simulink model "P702_NI_SoftECU"  (R2019a)
settings: Solver=ode1  StartTime=0.0  StopTime=Inf  FixedStep=0.001  RelTol=1e-3  EnableMultiTasking=on
PreLoadFcn:
  | run '.\VeriStand_BlockSet\NIVeriStandAddPaths.m'
undefined symbols (not defined in the file or in its folder): magnitude
libraries: simulink x83, simulink_extras x1
(part 74 of 76)

== system P702_NI_SoftECU/Output/Subsystem2/CAN_Signal/GWM/Other_GWMTx/Battery_Mgmt_24V_FD1 ==
  BattULo24Soc_Pc_Actl : Constant  Value=0
  BattULo24State_D_Qlty : Constant  Value=0
  BattULo24_Ah_DeltaRide : Constant  Value=0
  BattULo24_B_Falt : Constant  Value=0
  BattULo24_I_Actl : Constant  Value=0
  bus_creator : BusCreator  Inputs=5
  out_port : Outport
  wires:
  bus_creator/1 -> out_port/1  "Subsystem2"
  BattULo24Soc_Pc_Actl/1 -> bus_creator/1  "BattULo24Soc_Pc_Actl"
  BattULo24State_D_Qlty/1 -> bus_creator/2  "BattULo24State_D_Qlty"
  BattULo24_Ah_DeltaRide/1 -> bus_creator/3  "BattULo24_Ah_DeltaRide"
  BattULo24_B_Falt/1 -> bus_creator/4  "BattULo24_B_Falt"
  BattULo24_I_Actl/1 -> bus_creator/5  "BattULo24_I_Actl"

== system P702_NI_SoftECU/Output/Subsystem2/CAN_Signal/GWM/Other_GWMTx/Battery_Mgmt_2_FD1 ==
  BattULoChrg_D_Rq : Constant  Value=0
  BattULoSrvc_T_Actl : Constant  Value=0
  Batt_Crit_SoC_B : Constant  Value=0
  Batt_Lo_SoC_B : Constant  Value=0
  ChargeMode : Constant  Value=0
  EngStrtInhbt_B_RqBatt : Constant  Value=0
  IdleSpeedIncrease_El : Constant  Value=0
  PeriodicElLoad_B_Stat : Constant  Value=0
  PwSysULoFalt_D_Stat : Constant  Value=0
  Shed_Drain_Eng_Off_B : Constant  Value=0
  Shed_Feature_Group_ID : Constant  Value=0
  Shed_Level_Req : Constant  Value=0
  Shed_T_Eng_Off_B : Constant  Value=0
  ULoRgenTestMde_B_Rq : Constant  Value=0
  bus_creator : BusCreator  Inputs=14
  out_port : Outport
  wires:
  bus_creator/1 -> out_port/1  "Subsystem2"
  BattULoChrg_D_Rq/1 -> bus_creator/1  "BattULoChrg_D_Rq"
  BattULoSrvc_T_Actl/1 -> bus_creator/2  "BattULoSrvc_T_Actl"
  Batt_Crit_SoC_B/1 -> bus_creator/3  "Batt_Crit_SoC_B"
  Batt_Lo_SoC_B/1 -> bus_creator/4  "Batt_Lo_SoC_B"
  ChargeMode/1 -> bus_creator/5  "ChargeMode"
  EngStrtInhbt_B_RqBatt/1 -> bus_creator/6  "EngStrtInhbt_B_RqBatt"
  IdleSpeedIncrease_El/1 -> bus_creator/7  "IdleSpeedIncrease_El"
  PeriodicElLoad_B_Stat/1 -> bus_creator/8  "PeriodicElLoad_B_Stat"
  PwSysULoFalt_D_Stat/1 -> bus_creator/9  "PwSysULoFalt_D_Stat"
  Shed_Drain_Eng_Off_B/1 -> bus_creator/10  "Shed_Drain_Eng_Off_B"
  Shed_Feature_Group_ID/1 -> bus_creator/11  "Shed_Feature_Group_ID"
  Shed_Level_Req/1 -> bus_creator/12  "Shed_Level_Req"
  Shed_T_Eng_Off_B/1 -> bus_creator/13  "Shed_T_Eng_Off_B"
  ULoRgenTestMde_B_Rq/1 -> bus_creator/14  "ULoRgenTestMde_B_Rq"

== system P702_NI_SoftECU/Output/Subsystem2/CAN_Signal/GWM/Other_GWMTx/Battery_Mgmt_3_FD1 ==
  BSBattQCapAh : Constant  Value=0
  BSBattQDeltaRideAh : Constant  Value=0
  BSBattSOC : Constant  Value=0
  BSFault : Constant  Value=0
  BattULo2_Te_Actl : Constant  Value=0
  BattULoChrg_URate_RqMx : Constant  Value=0
  BattULoChrg_U_RqMn : Constant  Value=0
  BattULoChrg_U_RqMx : Constant  Value=0
  BattULoState_D_Qlty : Constant  Value=0
  bus_creator : BusCreator  Inputs=9
  out_port : Outport
  wires:
  bus_creator/1 -> out_port/1  "Subsystem2"
  BSBattQCapAh/1 -> bus_creator/1  "BSBattQCapAh"
  BSBattQDeltaRideAh/1 -> bus_creator/2  "BSBattQDeltaRideAh"
  BSBattSOC/1 -> bus_creator/3  "BSBattSOC"
  BSFault/1 -> bus_creator/4  "BSFault"
  BattULo2_Te_Actl/1 -> bus_creator/5  "BattULo2_Te_Actl"
  BattULoChrg_URate_RqMx/1 -> bus_creator/6  "BattULoChrg_URate_RqMx"
  BattULoChrg_U_RqMn/1 -> bus_creator/7  "BattULoChrg_U_RqMn"
  BattULoChrg_U_RqMx/1 -> bus_creator/8  "BattULoChrg_U_RqMx"
  BattULoState_D_Qlty/1 -> bus_creator/9  "BattULoState_D_Qlty"

== system P702_NI_SoftECU/Output/Subsystem2/CAN_Signal/GWM/Other_GWMTx/Battery_Mgmt_4_FD1 ==
  BattULoAuxSoc_Pc_Actl : Constant  Value=0
  BattULoAux_B_Falt : Constant  Value=0
  BattULoAux_D_Qlty : Constant  Value=0
  BattULoAux_I_Actl : Constant  Value=0
  BattULoAux_U_Actl : Constant  Value=0
  BattULoCrnkBelt_U_Pred : Constant  Value=0
  BattULoCrnkStrt_U_Pred : Constant  Value=0
  bus_creator : BusCreator  Inputs=7
  out_port : Outport
  wires:
  bus_creator/1 -> out_port/1  "Subsystem2"
  BattULoAuxSoc_Pc_Actl/1 -> bus_creator/1  "BattULoAuxSoc_Pc_Actl"
  BattULoAux_B_Falt/1 -> bus_creator/2  "BattULoAux_B_Falt"
  BattULoAux_D_Qlty/1 -> bus_creator/3  "BattULoAux_D_Qlty"
  BattULoAux_I_Actl/1 -> bus_creator/4  "BattULoAux_I_Actl"
  BattULoAux_U_Actl/1 -> bus_creator/5  "BattULoAux_U_Actl"
  BattULoCrnkBelt_U_Pred/1 -> bus_creator/6  "BattULoCrnkBelt_U_Pred"
  BattULoCrnkStrt_U_Pred/1 -> bus_creator/7  "BattULoCrnkStrt_U_Pred"

== system P702_NI_SoftECU/Output/Subsystem2/CAN_Signal/GWM/Other_GWMTx/Battery_Traction_1_FD1 ==
  BattTracMil_D_Rq : Constant  Value=0
  BattTracOffFst_D_Actl : Constant  Value=0
  BattTracOff_B_Actl : Constant  Value=0
  BattTrac_I_Actl : Constant  Value=0
  BattTrac_U_Actl : Constant  Value=0
  BattTrac_U_LimHi : Constant  Value=0
  BattTrac_U_LimLo : Constant  Value=0
  VehStrtInhbt_B_RqBatt : Constant  Value=0
  bus_creator : BusCreator  Inputs=8
  out_port : Outport
  wires:
  bus_creator/1 -> out_port/1  "Subsystem2"
  BattTracMil_D_Rq/1 -> bus_creator/1  "BattTracMil_D_Rq"
  BattTracOffFst_D_Actl/1 -> bus_creator/2  "BattTracOffFst_D_Actl"
  BattTracOff_B_Actl/1 -> bus_creator/3  "BattTracOff_B_Actl"
  BattTrac_I_Actl/1 -> bus_creator/4  "BattTrac_I_Actl"
  BattTrac_U_Actl/1 -> bus_creator/5  "BattTrac_U_Actl"
  BattTrac_U_LimHi/1 -> bus_creator/6  "BattTrac_U_LimHi"
  BattTrac_U_LimLo/1 -> bus_creator/7  "BattTrac_U_LimLo"
  VehStrtInhbt_B_RqBatt/1 -> bus_creator/8  "VehStrtInhbt_B_RqBatt"

== system P702_NI_SoftECU/Output/Subsystem2/CAN_Signal/GWM/Other_GWMTx/Battery_Traction_3_FD1 ==
  BattTracClnt_Te_Actl : Constant  Value=0
  BattTracSoc_Pc_LimHi : Constant  Value=0
  BattTracSoc_Pc_LimLo : Constant  Value=0
  BattTracSoc_Pc_MnPrtct : Constant  Value=0
  BattTracSoc_Pc_MxPrtct : Constant  Value=0
  BattTracSrvcRqd_B_Rq : Constant  Value=0
  BattTracWarnLamp_B_Rq : Constant  Value=0
  bus_creator : BusCreator  Inputs=7
  out_port : Outport
  wires:
  bus_creator/1 -> out_port/1  "Subsystem2"
  BattTracClnt_Te_Actl/1 -> bus_creator/1  "BattTracClnt_Te_Actl"
  BattTracSoc_Pc_LimHi/1 -> bus_creator/2  "BattTracSoc_Pc_LimHi"
  BattTracSoc_Pc_LimLo/1 -> bus_creator/3  "BattTracSoc_Pc_LimLo"
  BattTracSoc_Pc_MnPrtct/1 -> bus_creator/4  "BattTracSoc_Pc_MnPrtct"
  BattTracSoc_Pc_MxPrtct/1 -> bus_creator/5  "BattTracSoc_Pc_MxPrtct"
  BattTracSrvcRqd_B_Rq/1 -> bus_creator/6  "BattTracSrvcRqd_B_Rq"
  BattTracWarnLamp_B_Rq/1 -> bus_creator/7  "BattTracWarnLamp_B_Rq"

== system P702_NI_SoftECU/Output/Subsystem2/CAN_Signal/GWM/Other_GWMTx/Battery_Traction_4_FD1 ==
  BattTracDiagClr_B_Rq : Constant  Value=0
  BattTracSoc2_Pc_Actl : Constant  Value=0
  BattTrac_Te_Actl : Constant  Value=0
  bus_creator : BusCreator  Inputs=3
  out_port : Outport
  wires:
  bus_creator/1 -> out_port/1  "Subsystem2"
  BattTracDiagClr_B_Rq/1 -> bus_creator/1  "BattTracDiagClr_B_Rq"
  BattTracSoc2_Pc_Actl/1 -> bus_creator/2  "BattTracSoc2_Pc_Actl"
  BattTrac_Te_Actl/1 -> bus_creator/3  "BattTrac_Te_Actl"

== system P702_NI_SoftECU/Output/Subsystem2/CAN_Signal/GWM/Other_GWMTx/Battery_Traction_5_FD1 ==
  BattTrac2_Pw_ChrgInst : Constant  Value=0
  BattTrac2_Pw_DchrgInst : Constant  Value=0
  BattTrac2_Pw_LimChrg : Constant  Value=0
  BattTrac2_Pw_LimDchrg : Constant  Value=0
  bus_creator : BusCreator  Inputs=4
  out_port : Outport
  wires:
  bus_creator/1 -> out_port/1  "Subsystem2"
  BattTrac2_Pw_ChrgInst/1 -> bus_creator/1  "BattTrac2_Pw_ChrgInst"
  BattTrac2_Pw_DchrgInst/1 -> bus_creator/2  "BattTrac2_Pw_DchrgInst"
  BattTrac2_Pw_LimChrg/1 -> bus_creator/3  "BattTrac2_Pw_LimChrg"
  BattTrac2_Pw_LimDchrg/1 -> bus_creator/4  "BattTrac2_Pw_LimDchrg"

== system P702_NI_SoftECU/Output/Subsystem2/CAN_Signal/GWM/Other_GWMTx/Battery_Traction_6_FD1 ==
  BattTracClntPmp_D_Stat : Constant  Value=0
  BattTracCnnct_D_Cmd : Constant  Value=0
  BattTracDcdcDis_B_Rq : Constant  Value=0
  BattTracDelta_Te_Actl : Constant  Value=0
  BattTracHvilOpen_B_Stat : Constant  Value=0
  HtrnClntPump_D_Stat : Constant  Value=0
  bus_creator : BusCreator  Inputs=6
  out_port : Outport
  wires:
  bus_creator/1 -> out_port/1  "Subsystem2"
  BattTracClntPmp_D_Stat/1 -> bus_creator/1  "BattTracClntPmp_D_Stat"
  BattTracCnnct_D_Cmd/1 -> bus_creator/2  "BattTracCnnct_D_Cmd"
  BattTracDcdcDis_B_Rq/1 -> bus_creator/3  "BattTracDcdcDis_B_Rq"
  BattTracDelta_Te_Actl/1 -> bus_creator/4  "BattTracDelta_Te_Actl"
  BattTracHvilOpen_B_Stat/1 -> bus_creator/5  "BattTracHvilOpen_B_Stat"
  HtrnClntPump_D_Stat/1 -> bus_creator/6  "HtrnClntPump_D_Stat"

== system P702_NI_SoftECU/Output/Subsystem2/CAN_Signal/GWM/Other_GWMTx/BodyInfo_3_FD1 ==
  Backlit_LED_Status : Constant  Value=0
  BodySrvcRqd_B_Rq : Constant  Value=0
  CrashEvnt_D_Stat : Constant  Value=0
  Day_Night_Status : Constant  Value=0
  Delay_Accy : Constant  Value=0
  DimmingLvlEvnt_No_Actl : Constant  Value=0
  Dimming_Lvl : Constant  Value=0
  DrStatDrvErrCnt_B_Stat : Constant  Value=0
  DrStatDrv_B_Actl : Constant  Value=0
  DrStatHood_B_Actl : Constant  Value=0
  DrStatInnrTgate_B_Actl : Constant  Value=0
  DrStatPsngr_B_Actl : Constant  Value=0
  DrStatRl_B_Actl : Constant  Value=0
  DrStatRr_B_Actl : Constant  Value=0
  DrStatTgate_B_Actl : Constant  Value=0
  FogLghtFrontOn_B_Stat : Constant  Value=0
  FogLghtRearOn_B_Stat : Constant  Value=0
  FuelPmpInhbt_B_Stat : Constant  Value=0
  IgnKeyType_D_Actl : Constant  Value=0
  Ignition_Status : Constant  Value=0
  Key_In_Ignition_Stat : Constant  Value=0
  LifeCycMde_D_Actl : Constant  Value=0
  Litval : Constant  Value=0
  Parklamp_Status : Constant  Value=0
  PrkBrkActv_B_Actl : Constant  Value=0
  Remote_Start_Status : Constant  Value=0
  TurnLghtLeftOn_B_Stat : Constant  Value=0
  TurnLghtLeft_D_Rq : Constant  Value=0
  TurnLghtRightOn_B_Stat : Constant  Value=0
  TurnLghtRight_D_Rq : Constant  Value=0
  ValetMode_D_Mem : Constant  Value=0
  bus_creator : BusCreator  Inputs=31
  out_port : Outport
  wires:
  bus_creator/1 -> out_port/1  "Subsystem2"
  Backlit_LED_Status/1 -> bus_creator/1  "Backlit_LED_Status"
  BodySrvcRqd_B_Rq/1 -> bus_creator/2  "BodySrvcRqd_B_Rq"
  CrashEvnt_D_Stat/1 -> bus_creator/3  "CrashEvnt_D_Stat"
  Day_Night_Status/1 -> bus_creator/4  "Day_Night_Status"
  Delay_Accy/1 -> bus_creator/5  "Delay_Accy"
  DimmingLvlEvnt_No_Actl/1 -> bus_creator/6  "DimmingLvlEvnt_No_Actl"
  Dimming_Lvl/1 -> bus_creator/7  "Dimming_Lvl"
  DrStatDrvErrCnt_B_Stat/1 -> bus_creator/8  "DrStatDrvErrCnt_B_Stat"
  DrStatDrv_B_Actl/1 -> bus_creator/9  "DrStatDrv_B_Actl"
  DrStatHood_B_Actl/1 -> bus_creator/10  "DrStatHood_B_Actl"
  DrStatInnrTgate_B_Actl/1 -> bus_creator/11  "DrStatInnrTgate_B_Actl"
  DrStatPsngr_B_Actl/1 -> bus_creator/12  "DrStatPsngr_B_Actl"
  DrStatRl_B_Actl/1 -> bus_creator/13  "DrStatRl_B_Actl"
  DrStatRr_B_Actl/1 -> bus_creator/14  "DrStatRr_B_Actl"
  DrStatTgate_B_Actl/1 -> bus_creator/15  "DrStatTgate_B_Actl"
  FogLghtFrontOn_B_Stat/1 -> bus_creator/16  "FogLghtFrontOn_B_Stat"
  FogLghtRearOn_B_Stat/1 -> bus_creator/17  "FogLghtRearOn_B_Stat"
  FuelPmpInhbt_B_Stat/1 -> bus_creator/18  "FuelPmpInhbt_B_Stat"
  IgnKeyType_D_Actl/1 -> bus_creator/19  "IgnKeyType_D_Actl"
  Ignition_Status/1 -> bus_creator/20  "Ignition_Status"
  Key_In_Ignition_Stat/1 -> bus_creator/21  "Key_In_Ignition_Stat"
  LifeCycMde_D_Actl/1 -> bus_creator/22  "LifeCycMde_D_Actl"
  Litval/1 -> bus_creator/23  "Litval"
  Parklamp_Status/1 -> bus_creator/24  "Parklamp_Status"
  PrkBrkActv_B_Actl/1 -> bus_creator/25  "PrkBrkActv_B_Actl"
  Remote_Start_Status/1 -> bus_creator/26  "Remote_Start_Status"
  TurnLghtLeftOn_B_Stat/1 -> bus_creator/27  "TurnLghtLeftOn_B_Stat"
  TurnLghtLeft_D_Rq/1 -> bus_creator/28  "TurnLghtLeft_D_Rq"
  TurnLghtRightOn_B_Stat/1 -> bus_creator/29  "TurnLghtRightOn_B_Stat"
  TurnLghtRight_D_Rq/1 -> bus_creator/30  "TurnLghtRight_D_Rq"
  ValetMode_D_Mem/1 -> bus_creator/31  "ValetMode_D_Mem"

== system P702_NI_SoftECU/Output/Subsystem2/CAN_Signal/GWM/Other_GWMTx/Body_Info_10_FD1 ==
  GenericSwtch1_No_Actl : Constant  Value=0
  GenericSwtch2_No_Actl : Constant  Value=0
  GenericSwtch3_No_Actl : Constant  Value=0
  bus_creator : BusCreator  Inputs=3
  out_port : Outport
  wires:
  bus_creator/1 -> out_port/1  "Subsystem2"
  GenericSwtch1_No_Actl/1 -> bus_creator/1  "GenericSwtch1_No_Actl"
  GenericSwtch2_No_Actl/1 -> bus_creator/2  "GenericSwtch2_No_Actl"
  GenericSwtch3_No_Actl/1 -> bus_creator/3  "GenericSwtch3_No_Actl"

== system P702_NI_SoftECU/Output/Subsystem2/CAN_Signal/GWM/Other_GWMTx/Body_Info_4_FD1 ==
  BattULo_I_Actl : Constant  Value=0
  BattULo_U_Actl : Constant  Value=0
  BrkTrnShifLck_B_Stat : Constant  Value=0
  DcacElPw_D_Rq : Constant  Value=0
  DriverCrankingReq : Constant  Value=0
  EngOff_T_Actl : Constant  Value=0
  FuelPumpPwr_D_Stat : Constant  Value=0
  PrkLckCtlAvail_T_Stat : Constant  Value=0
  PrkLckCtlMsgTxt_D_Rq : Constant  Value=0
  PrkLckCtlTow_B_Enbl : Constant  Value=0
  PrkLckCtlUnlck_D_Stat : Constant  Value=0
  PrkLckCtl_B_Enbl : Constant  Value=0
  PtLatchActv_B_RqBcm : Constant  Value=0
  ReFuelSwtchStat_D_Actl : Constant  Value=0
  bus_creator : BusCreator  Inputs=15
  immoSecureIdleMode : Constant  Value=0
  out_port : Outport
  wires:
  bus_creator/1 -> out_port/1  "Subsystem2"
  BattULo_I_Actl/1 -> bus_creator/1  "BattULo_I_Actl"
  BattULo_U_Actl/1 -> bus_creator/2  "BattULo_U_Actl"
  BrkTrnShifLck_B_Stat/1 -> bus_creator/3  "BrkTrnShifLck_B_Stat"
  DcacElPw_D_Rq/1 -> bus_creator/4  "DcacElPw_D_Rq"
  DriverCrankingReq/1 -> bus_creator/5  "DriverCrankingReq"
  EngOff_T_Actl/1 -> bus_creator/6  "EngOff_T_Actl"
  FuelPumpPwr_D_Stat/1 -> bus_creator/7  "FuelPumpPwr_D_Stat"
  PrkLckCtlAvail_T_Stat/1 -> bus_creator/8  "PrkLckCtlAvail_T_Stat"
  PrkLckCtlMsgTxt_D_Rq/1 -> bus_creator/9  "PrkLckCtlMsgTxt_D_Rq"
  PrkLckCtlTow_B_Enbl/1 -> bus_creator/10  "PrkLckCtlTow_B_Enbl"
  PrkLckCtlUnlck_D_Stat/1 -> bus_creator/11  "PrkLckCtlUnlck_D_Stat"
  PrkLckCtl_B_Enbl/1 -> bus_creator/12  "PrkLckCtl_B_Enbl"
  PtLatchActv_B_RqBcm/1 -> bus_creator/13  "PtLatchActv_B_RqBcm"
  ReFuelSwtchStat_D_Actl/1 -> bus_creator/14  "ReFuelSwtchStat_D_Actl"
  immoSecureIdleMode/1 -> bus_creator/15  "immoSecureIdleMode"

== system P702_NI_SoftECU/Output/Subsystem2/CAN_Signal/GWM/Other_GWMTx/Body_Info_6_FD1 ==
  DrLatchMsgTxt_D_Rq : Constant  Value=0
  ElPwPoint_D_Rq : Constant  Value=0
  HeadLghtHiPrmsn_D_Stat : Constant  Value=0
  IgnPsswrdDsply_B_Rq : Constant  Value=0
  KeyAdmnTot_No_Cnt : Constant  Value=0
  KeyMykeyTot_No_Cnt : Constant  Value=0
  Keycode_Status : Constant  Value=0
  PEBackupSlot_Stats : Constant  Value=0
  PoliceIdlMde_D_Stat : Constant  Value=0
  PrmtrAlrmEvnt_D_Stat : Constant  Value=0
  PrsnlDevcChrgEnbl_B_Rq : Constant  Value=0
  SecurityMsgTxt_D_Rq : Constant  Value=0
  SteWhlLckMsgTxt_D_Rq : Constant  Value=0
  TracKeyMde_D_Stat : Constant  Value=0
  bus_creator : BusCreator  Inputs=15
  immoMsgTxt_D_Rq : Constant  Value=0
  out_port : Outport
  wires:
  bus_creator/1 -> out_port/1  "Subsystem2"
  DrLatchMsgTxt_D_Rq/1 -> bus_creator/1  "DrLatchMsgTxt_D_Rq"
  ElPwPoint_D_Rq/1 -> bus_creator/2  "ElPwPoint_D_Rq"
  HeadLghtHiPrmsn_D_Stat/1 -> bus_creator/3  "HeadLghtHiPrmsn_D_Stat"
  IgnPsswrdDsply_B_Rq/1 -> bus_creator/4  "IgnPsswrdDsply_B_Rq"
  KeyAdmnTot_No_Cnt/1 -> bus_creator/5  "KeyAdmnTot_No_Cnt"
  KeyMykeyTot_No_Cnt/1 -> bus_creator/6  "KeyMykeyTot_No_Cnt"
  Keycode_Status/1 -> bus_creator/7  "Keycode_Status"
  PEBackupSlot_Stats/1 -> bus_creator/8  "PEBackupSlot_Stats"
  PoliceIdlMde_D_Stat/1 -> bus_creator/9  "PoliceIdlMde_D_Stat"
  PrmtrAlrmEvnt_D_Stat/1 -> bus_creator/10  "PrmtrAlrmEvnt_D_Stat"
  PrsnlDevcChrgEnbl_B_Rq/1 -> bus_creator/11  "PrsnlDevcChrgEnbl_B_Rq"
  SecurityMsgTxt_D_Rq/1 -> bus_creator/12  "SecurityMsgTxt_D_Rq"
  SteWhlLckMsgTxt_D_Rq/1 -> bus_creator/13  "SteWhlLckMsgTxt_D_Rq"
  TracKeyMde_D_Stat/1 -> bus_creator/14  "TracKeyMde_D_Stat"
  immoMsgTxt_D_Rq/1 -> bus_creator/15  "immoMsgTxt_D_Rq"

== system P702_NI_SoftECU/Output/Subsystem2/CAN_Signal/GWM/Other_GWMTx/Body_Info_8_FD1 ==
  ChrgCordLck_B_Stat : Constant  Value=0
  ChrgCordResp1_No_Actl : Constant  Value=0
  ChrgCordResp2_No_Actl : Constant  Value=0
  WakeAlarm0_D_Stat : Constant  Value=0
  WakeAlarm1_D_Stat : Constant  Value=0
  WakeAlarm2_D_Stat : Constant  Value=0
  WakeAlarm3_D_Stat : Constant  Value=0
  bus_creator : BusCreator  Inputs=7
  out_port : Outport
  wires:
  bus_creator/1 -> out_port/1  "Subsystem2"
  ChrgCordLck_B_Stat/1 -> bus_creator/1  "ChrgCordLck_B_Stat"
  ChrgCordResp1_No_Actl/1 -> bus_creator/2  "ChrgCordResp1_No_Actl"
  ChrgCordResp2_No_Actl/1 -> bus_creator/3  "ChrgCordResp2_No_Actl"
  WakeAlarm0_D_Stat/1 -> bus_creator/4  "WakeAlarm0_D_Stat"
  WakeAlarm1_D_Stat/1 -> bus_creator/5  "WakeAlarm1_D_Stat"
  WakeAlarm2_D_Stat/1 -> bus_creator/6  "WakeAlarm2_D_Stat"
  WakeAlarm3_D_Stat/1 -> bus_creator/7  "WakeAlarm3_D_Stat"

== system P702_NI_SoftECU/Output/Subsystem2/CAN_Signal/GWM/Other_GWMTx/Body_Info_9_FD1 ==
  AdvStrt_D_Stat : Constant  Value=0
  CrnkInhbt_B_Stat : Constant  Value=0
  CrnkInhbt_No_Cnt : Constant  Value=0
  CrnkInhbt_No_Cs : Constant  Value=0
  DrvInCtl_B_Stat : Constant  Value=0
  EngStrtActv_B_Stat : Constant  Value=0
  EngStrt_B_Rq : Constant  Value=0
  IgnPreOffActv_B_Stat : Constant  Value=0
  StrtrMtrCtlDStat_No_Cs : Constant  Value=0
  VehOnSrc_D_Stat : Constant  Value=0
  bus_creator : BusCreator  Inputs=10
  out_port : Outport
  wires:
  bus_creator/1 -> out_port/1  "Subsystem2"
  AdvStrt_D_Stat/1 -> bus_creator/1  "AdvStrt_D_Stat"
  CrnkInhbt_B_Stat/1 -> bus_creator/2  "CrnkInhbt_B_Stat"
  CrnkInhbt_No_Cnt/1 -> bus_creator/3  "CrnkInhbt_No_Cnt"
  CrnkInhbt_No_Cs/1 -> bus_creator/4  "CrnkInhbt_No_Cs"
  DrvInCtl_B_Stat/1 -> bus_creator/5  "DrvInCtl_B_Stat"
  EngStrtActv_B_Stat/1 -> bus_creator/6  "EngStrtActv_B_Stat"
  EngStrt_B_Rq/1 -> bus_creator/7  "EngStrt_B_Rq"
  IgnPreOffActv_B_Stat/1 -> bus_creator/8  "IgnPreOffActv_B_Stat"
  StrtrMtrCtlDStat_No_Cs/1 -> bus_creator/9  "StrtrMtrCtlDStat_No_Cs"
  VehOnSrc_D_Stat/1 -> bus_creator/10  "VehOnSrc_D_Stat"

== system P702_NI_SoftECU/Output/Subsystem2/CAN_Signal/GWM/Other_GWMTx/Climate_Cntrl_Data_2_FD1 ==
  ApaSwtch_D_RqDrv : Constant  Value=0
  ApaSwtch_No_Cnt : Constant  Value=0
  CabnAmb_Te_Actl : Constant  Value=0
  CamraDefog_B_Actl : Constant  Value=0
  ClimtThrmlLoad_No_Actl : Constant  Value=0
  EcoMde_D_RqDrv : Constant  Value=0
  HvacAir_Flw_Est : Constant  Value=0
  HvacBlwrFront_D_Stat : Constant  Value=0
  HvacBlwrRear_D_Stat : Constant  Value=0
  HvacRec_Pc_Est : Constant  Value=0
  HvacRemoteStrt_N_Rq : Constant  Value=0
  TwHlGrdAsst_B_RqTrn : Constant  Value=0
  bus_creator : BusCreator  Inputs=12
  out_port : Outport
  wires:
  bus_creator/1 -> out_port/1  "Subsystem2"
  ApaSwtch_D_RqDrv/1 -> bus_creator/1  "ApaSwtch_D_RqDrv"
  ApaSwtch_No_Cnt/1 -> bus_creator/2  "ApaSwtch_No_Cnt"
  CabnAmb_Te_Actl/1 -> bus_creator/3  "CabnAmb_Te_Actl"
  CamraDefog_B_Actl/1 -> bus_creator/4  "CamraDefog_B_Actl"
  ClimtThrmlLoad_No_Actl/1 -> bus_creator/5  "ClimtThrmlLoad_No_Actl"
  EcoMde_D_RqDrv/1 -> bus_creator/6  "EcoMde_D_RqDrv"
  HvacAir_Flw_Est/1 -> bus_creator/7  "HvacAir_Flw_Est"
  HvacBlwrFront_D_Stat/1 -> bus_creator/8  "HvacBlwrFront_D_Stat"
  HvacBlwrRear_D_Stat/1 -> bus_creator/9  "HvacBlwrRear_D_Stat"
  HvacRec_Pc_Est/1 -> bus_creator/10  "HvacRec_Pc_Est"
  HvacRemoteStrt_N_Rq/1 -> bus_creator/11  "HvacRemoteStrt_N_Rq"
  TwHlGrdAsst_B_RqTrn/1 -> bus_creator/12  "TwHlGrdAsst_B_RqTrn"

== system P702_NI_SoftECU/Output/Subsystem2/CAN_Signal/GWM/Other_GWMTx/Climate_Control_Data_FD1 ==
  AutoHoldSwtch_D_Stat : Constant  Value=0
  CamraFrntBttn_D_Stat : Constant  Value=0
  CamraRearBttn_D_Stat : Constant  Value=0
  DrvSlipCtlMde_B_Rq : Constant  Value=0
  EcoInhbt_B_RqHvac : Constant  Value=0
  GlvBoxRleas_No_Actl : Constant  Value=0
  LpdbAuxBlwr_B_Rq : Constant  Value=0
  LpdbDfrstFlOn_B_Rq : Constant  Value=0
  LpdbDfrstFrOn_B_Rq : Constant  Value=0
  LpdbDfrstRearOn_B_Rq : Constant  Value=0
  LpdbHeatWiprPrk_B_Rq : Constant  Value=0
  LpdbPtc1_B_Rq : Constant  Value=0
  LpdbPtc2_B_Rq : Constant  Value=0
  LpdbPtc3_B_Rq : Constant  Value=0
  MirrorHeatOn_B_Rq : Constant  Value=0
  Outside_Air_Temp_Stat : Constant  Value=0
  PrkAidSwtch_D_RqDrv : Constant  Value=0
  PrkAidSwtch_No_Cnt : Constant  Value=0
  Remote_Start_QuietMode : Constant  Value=0
  SteWhlHeat_D_Rq : Constant  Value=0
  TrailCtlSwtch_B_Stat : Constant  Value=0
  bus_creator : BusCreator  Inputs=21
  out_port : Outport
  wires:
  bus_creator/1 -> out_port/1  "Subsystem2"
  AutoHoldSwtch_D_Stat/1 -> bus_creator/1  "AutoHoldSwtch_D_Stat"
  CamraFrntBttn_D_Stat/1 -> bus_creator/2  "CamraFrntBttn_D_Stat"
  CamraRearBttn_D_Stat/1 -> bus_creator/3  "CamraRearBttn_D_Stat"
  DrvSlipCtlMde_B_Rq/1 -> bus_creator/4  "DrvSlipCtlMde_B_Rq"
  EcoInhbt_B_RqHvac/1 -> bus_creator/5  "EcoInhbt_B_RqHvac"
  GlvBoxRleas_No_Actl/1 -> bus_creator/6  "GlvBoxRleas_No_Actl"
  LpdbAuxBlwr_B_Rq/1 -> bus_creator/7  "LpdbAuxBlwr_B_Rq"
  LpdbDfrstFlOn_B_Rq/1 -> bus_creator/8  "LpdbDfrstFlOn_B_Rq"
  LpdbDfrstFrOn_B_Rq/1 -> bus_creator/9  "LpdbDfrstFrOn_B_Rq"
  LpdbDfrstRearOn_B_Rq/1 -> bus_creator/10  "LpdbDfrstRearOn_B_Rq"
  LpdbHeatWiprPrk_B_Rq/1 -> bus_creator/11  "LpdbHeatWiprPrk_B_Rq"
  LpdbPtc1_B_Rq/1 -> bus_creator/12  "LpdbPtc1_B_Rq"
  LpdbPtc2_B_Rq/1 -> bus_creator/13  "LpdbPtc2_B_Rq"
  LpdbPtc3_B_Rq/1 -> bus_creator/14  "LpdbPtc3_B_Rq"
  MirrorHeatOn_B_Rq/1 -> bus_creator/15  "MirrorHeatOn_B_Rq"
  Outside_Air_Temp_Stat/1 -> bus_creator/16  "Outside_Air_Temp_Stat"
  PrkAidSwtch_D_RqDrv/1 -> bus_creator/17  "PrkAidSwtch_D_RqDrv"
  PrkAidSwtch_No_Cnt/1 -> bus_creator/18  "PrkAidSwtch_No_Cnt"
  Remote_Start_QuietMode/1 -> bus_creator/19  "Remote_Start_QuietMode"
  SteWhlHeat_D_Rq/1 -> bus_creator/20  "SteWhlHeat_D_Rq"
  TrailCtlSwtch_B_Stat/1 -> bus_creator/21  "TrailCtlSwtch_B_Stat"

== system P702_NI_SoftECU/Output/Subsystem2/CAN_Signal/GWM/Other_GWMTx/Cluster_Info1_FD1 ==
  AccDeny_B_RqIpc : Constant  Value=0
  AccEnbl_B_RqDrv : Constant  Value=0
  BulbChkActv_B_Stat : Constant  Value=0
  DrvPerfMde_D_Rq : Constant  Value=0
  DrvSlipCtlMde_B_Rq2 : Constant  Value=0
  DrvSlipCtlMde_D_Rq : Constant  Value=0
  EmgcyCallAsstMykey_Rq : Constant  Value=0
  EngIdlShutDown_B_RqDrv : Constant  Value=0
  EngOilLife_B_RqReset : Constant  Value=0
  Fda_B_Stat : Constant  Value=0
  FrostWarn_D_Stat : Constant  Value=0
  HsaMde_D_Rq : Constant  Value=0
  KeyTypeChngMykey_D_Rq : Constant  Value=0
  LscmbbStat_B_Actl : Constant  Value=0
  ManRgen_D_Rq : Constant  Value=0
  MetricActvTe_B_Actl : Constant  Value=0
  MetricActv_B_Actl : Constant  Value=0
  NtrlTowMdeEnbl_B_RqDrv : Constant  Value=0
  OdometerMasterValue : Constant  Value=0
  ParkDetect_Stat : Constant  Value=0
  Power_Liftgate_Mode_Cmd : Constant  Value=0
  PrkLckCtlEnbl_D_RqIpc : Constant  Value=0
  PtDrvMde_D_Rq : Constant  Value=0
  ReducedGuard_D_Rq : Constant  Value=0
  StopStrtDrvMde_D_RqMnu : Constant  Value=0
  TRAILER_BRAKE_CONFIG : Constant  Value=0
  TRLR_SWAY_CONFIG_CMD : Constant  Value=0
  TrlrBrkMde_D_Rq : Constant  Value=0
  bus_creator : BusCreator  Inputs=29
  ePRNDL_MODE : Constant  Value=0
  out_port : Outport
  wires:
  bus_creator/1 -> out_port/1  "Subsystem2"
  AccDeny_B_RqIpc/1 -> bus_creator/1  "AccDeny_B_RqIpc"
  AccEnbl_B_RqDrv/1 -> bus_creator/2  "AccEnbl_B_RqDrv"
  BulbChkActv_B_Stat/1 -> bus_creator/3  "BulbChkActv_B_Stat"
  DrvPerfMde_D_Rq/1 -> bus_creator/4  "DrvPerfMde_D_Rq"
  DrvSlipCtlMde_B_Rq2/1 -> bus_creator/5  "DrvSlipCtlMde_B_Rq2"
  DrvSlipCtlMde_D_Rq/1 -> bus_creator/6  "DrvSlipCtlMde_D_Rq"
  EmgcyCallAsstMykey_Rq/1 -> bus_creator/7  "EmgcyCallAsstMykey_Rq"
  EngIdlShutDown_B_RqDrv/1 -> bus_creator/8  "EngIdlShutDown_B_RqDrv"
  EngOilLife_B_RqReset/1 -> bus_creator/9  "EngOilLife_B_RqReset"
  Fda_B_Stat/1 -> bus_creator/10  "Fda_B_Stat"
  FrostWarn_D_Stat/1 -> bus_creator/11  "FrostWarn_D_Stat"
  HsaMde_D_Rq/1 -> bus_creator/12  "HsaMde_D_Rq"
  KeyTypeChngMykey_D_Rq/1 -> bus_creator/13  "KeyTypeChngMykey_D_Rq"
  LscmbbStat_B_Actl/1 -> bus_creator/14  "LscmbbStat_B_Actl"
  ManRgen_D_Rq/1 -> bus_creator/15  "ManRgen_D_Rq"
  MetricActvTe_B_Actl/1 -> bus_creator/16  "MetricActvTe_B_Actl"
  MetricActv_B_Actl/1 -> bus_creator/17  "MetricActv_B_Actl"
  NtrlTowMdeEnbl_B_RqDrv/1 -> bus_creator/18  "NtrlTowMdeEnbl_B_RqDrv"
  OdometerMasterValue/1 -> bus_creator/19  "OdometerMasterValue"
  ParkDetect_Stat/1 -> bus_creator/20  "ParkDetect_Stat"
  Power_Liftgate_Mode_Cmd/1 -> bus_creator/21  "Power_Liftgate_Mode_Cmd"
  PrkLckCtlEnbl_D_RqIpc/1 -> bus_creator/22  "PrkLckCtlEnbl_D_RqIpc"
  PtDrvMde_D_Rq/1 -> bus_creator/23  "PtDrvMde_D_Rq"
  ReducedGuard_D_Rq/1 -> bus_creator/24  "ReducedGuard_D_Rq"
  StopStrtDrvMde_D_RqMnu/1 -> bus_creator/25  "StopStrtDrvMde_D_RqMnu"
  TRAILER_BRAKE_CONFIG/1 -> bus_creator/26  "TRAILER_BRAKE_CONFIG"
  TRLR_SWAY_CONFIG_CMD/1 -> bus_creator/27  "TRLR_SWAY_CONFIG_CMD"
  TrlrBrkMde_D_Rq/1 -> bus_creator/28  "TrlrBrkMde_D_Rq"
  ePRNDL_MODE/1 -> bus_creator/29  "ePRNDL_MODE"

== system P702_NI_SoftECU/Output/Subsystem2/CAN_Signal/GWM/Other_GWMTx/Cluster_Info_3_FD1 ==
  AutoRgen_D_Rq : Constant  Value=0
  DISPLAY_SPEED_OFFSET : Constant  Value=0
  DISPLAY_SPEED_SCALING : Constant  Value=0
  DrvSlipCtlMde_B_RqMyKey : Constant  Value=0
  FUEL_SENSOR_NUM : Constant  Value=0
  FuelLvlActvSide_No_Raw : Constant  Value=0
  FuelLvlPssvSide_No_Raw : Constant  Value=0
  FuelLvlWarn_D_Actl : Constant  Value=0
  FuelLvl_Pc_Dsply : Constant  Value=0
  FuelSecndActv_B_Actl : Constant  Value=0
  OdoTripRx_B_Actl : Constant  Value=0
  Veh_V_CompLimMx : Constant  Value=0
  W2S_LAMP_OK : Constant  Value=0
  bus_creator : BusCreator  Inputs=13
  out_port : Outport
  wires:
  bus_creator/1 -> out_port/1  "Subsystem2"
  AutoRgen_D_Rq/1 -> bus_creator/1  "AutoRgen_D_Rq"
  DISPLAY_SPEED_OFFSET/1 -> bus_creator/2  "DISPLAY_SPEED_OFFSET"
  DISPLAY_SPEED_SCALING/1 -> bus_creator/3  "DISPLAY_SPEED_SCALING"
  DrvSlipCtlMde_B_RqMyKey/1 -> bus_creator/4  "DrvSlipCtlMde_B_RqMyKey"
  FUEL_SENSOR_NUM/1 -> bus_creator/5  "FUEL_SENSOR_NUM"
  FuelLvlActvSide_No_Raw/1 -> bus_creator/6  "FuelLvlActvSide_No_Raw"
  FuelLvlPssvSide_No_Raw/1 -> bus_creator/7  "FuelLvlPssvSide_No_Raw"
  FuelLvlWarn_D_Actl/1 -> bus_creator/8  "FuelLvlWarn_D_Actl"
  FuelLvl_Pc_Dsply/1 -> bus_creator/9  "FuelLvl_Pc_Dsply"
  FuelSecndActv_B_Actl/1 -> bus_creator/10  "FuelSecndActv_B_Actl"
  OdoTripRx_B_Actl/1 -> bus_creator/11  "OdoTripRx_B_Actl"
  Veh_V_CompLimMx/1 -> bus_creator/12  "Veh_V_CompLimMx"
  W2S_LAMP_OK/1 -> bus_creator/13  "W2S_LAMP_OK"

== system P702_NI_SoftECU/Output/Subsystem2/CAN_Signal/GWM/Other_GWMTx/Cluster_Lighting_Rq_FD1 ==
  IsaOffst_D_Rq : Constant  Value=0
  SlMde_D_Rq : Constant  Value=0
  bus_creator : BusCreator  Inputs=2
  out_port : Outport
  wires:
  bus_creator/1 -> out_port/1  "Subsystem2"
  IsaOffst_D_Rq/1 -> bus_creator/1  "IsaOffst_D_Rq"
  SlMde_D_Rq/1 -> bus_creator/2  "SlMde_D_Rq"

== system P702_NI_SoftECU/Output/Subsystem2/CAN_Signal/GWM/Other_GWMTx/Compressor_Req_FD1 ==
  ClimtCoolRear_B_Rq : Constant  Value=0
  ClimtCool_D_Rq : Constant  Value=0
  ClimtDeltaLoad_Pw_Actl : Constant  Value=0
  ClimtHeatRear_D_Rq : Constant  Value=0
  ClimtHeat_D_Rq : Constant  Value=0
  ClimtPw_B_Rq : Constant  Value=0
  HtrCorePump_B_Rq : Constant  Value=0
  HvacAirCond_B_Rq : Constant  Value=0
  HvacEvap_Te_Actl : Constant  Value=0
  HvacEvap_Te_Offst : Constant  Value=0
  HvacEvap_Te_Rq : Constant  Value=0
  HvacHtrCore_Te_Rq : Constant  Value=0
  SnowPlowMde_B_Enbl : Constant  Value=0
  StopStrtDrvMde_B_RqBtn : Constant  Value=0
  WndwFrontHeat_B_Stat : Constant  Value=0
  bus_creator : BusCreator  Inputs=15
  out_port : Outport
  wires:
  bus_creator/1 -> out_port/1  "Subsystem2"
  ClimtCoolRear_B_Rq/1 -> bus_creator/1  "ClimtCoolRear_B_Rq"
  ClimtCool_D_Rq/1 -> bus_creator/2  "ClimtCool_D_Rq"
  ClimtDeltaLoad_Pw_Actl/1 -> bus_creator/3  "ClimtDeltaLoad_Pw_Actl"
  ClimtHeatRear_D_Rq/1 -> bus_creator/4  "ClimtHeatRear_D_Rq"
  ClimtHeat_D_Rq/1 -> bus_creator/5  "ClimtHeat_D_Rq"
  ClimtPw_B_Rq/1 -> bus_creator/6  "ClimtPw_B_Rq"
  HtrCorePump_B_Rq/1 -> bus_creator/7  "HtrCorePump_B_Rq"
  HvacAirCond_B_Rq/1 -> bus_creator/8  "HvacAirCond_B_Rq"
  HvacEvap_Te_Actl/1 -> bus_creator/9  "HvacEvap_Te_Actl"
  HvacEvap_Te_Offst/1 -> bus_creator/10  "HvacEvap_Te_Offst"
  HvacEvap_Te_Rq/1 -> bus_creator/11  "HvacEvap_Te_Rq"
  HvacHtrCore_Te_Rq/1 -> bus_creator/12  "HvacHtrCore_Te_Rq"
  SnowPlowMde_B_Enbl/1 -> bus_creator/13  "SnowPlowMde_B_Enbl"
  StopStrtDrvMde_B_RqBtn/1 -> bus_creator/14  "StopStrtDrvMde_B_RqBtn"
  WndwFrontHeat_B_Stat/1 -> bus_creator/15  "WndwFrontHeat_B_Stat"

== system P702_NI_SoftECU/Output/Subsystem2/CAN_Signal/GWM/Other_GWMTx/CruiseCtrl_Strg_Data_FD1 ==
  AccButtnGapDecPress2 : Constant  Value=0
  AccButtnGapIncPress2 : Constant  Value=0
  AccButtnGpTogglePress2 : Constant  Value=0
  ActvFrontSteLck_D_Stat : Constant  Value=0
  ActvFrontSteMsgTxt_D_Rq : Constant  Value=0
  AslButtnOnOffCnclPres2 : Constant  Value=0
  AslButtnOnOffPress2 : Constant  Value=0
  CcAslButtnCnclPress2 : Constant  Value=0
  CcAslButtnCnclResPres2 : Constant  Value=0
  CcAslButtnDeny_B_Actl2 : Constant  Value=0
  CcAslButtnIndxDecPres2 : Constant  Value=0
  CcAslButtnIndxIncPres2 : Constant  Value=0
  CcAslButtnOffCnclPres2 : Constant  Value=0
  CcAslButtnOnOffCncl2 : Constant  Value=0
  CcAslButtnOnPress2 : Constant  Value=0
  CcAslButtnResDecPress2 : Constant  Value=0
  CcAslButtnResIncPress2 : Constant  Value=0
  CcAslButtnSetDecPress2 : Constant  Value=0
  CcAslButtnSetIncPress2 : Constant  Value=0
  CcAslButtnSetPress2 : Constant  Value=0
  CcAsllButtnResPress2 : Constant  Value=0
  CcButtnOffPress2 : Constant  Value=0
  CcButtnOnOffCnclPress2 : Constant  Value=0
  CcButtnOnOffPress2 : Constant  Value=0
  CcButtnOnPress2 : Constant  Value=0
  SelDrvMdeAdptSte_D_Stat : Constant  Value=0
  TjaButtnOnOffPress2 : Constant  Value=0
  bus_creator : BusCreator  Inputs=27
  out_port : Outport
  wires:
  bus_creator/1 -> out_port/1  "Subsystem2"
  AccButtnGapDecPress2/1 -> bus_creator/1  "AccButtnGapDecPress2"
  AccButtnGapIncPress2/1 -> bus_creator/2  "AccButtnGapIncPress2"
  AccButtnGpTogglePress2/1 -> bus_creator/3  "AccButtnGpTogglePress2"
  ActvFrontSteLck_D_Stat/1 -> bus_creator/4  "ActvFrontSteLck_D_Stat"
  ActvFrontSteMsgTxt_D_Rq/1 -> bus_creator/5  "ActvFrontSteMsgTxt_D_Rq"
  AslButtnOnOffCnclPres2/1 -> bus_creator/6  "AslButtnOnOffCnclPres2"
  AslButtnOnOffPress2/1 -> bus_creator/7  "AslButtnOnOffPress2"
  CcAslButtnCnclPress2/1 -> bus_creator/8  "CcAslButtnCnclPress2"
  CcAslButtnCnclResPres2/1 -> bus_creator/9  "CcAslButtnCnclResPres2"
  CcAslButtnDeny_B_Actl2/1 -> bus_creator/10  "CcAslButtnDeny_B_Actl2"
  CcAslButtnIndxDecPres2/1 -> bus_creator/11  "CcAslButtnIndxDecPres2"
  CcAslButtnIndxIncPres2/1 -> bus_creator/12  "CcAslButtnIndxIncPres2"
  CcAslButtnOffCnclPres2/1 -> bus_creator/13  "CcAslButtnOffCnclPres2"
  CcAslButtnOnOffCncl2/1 -> bus_creator/14  "CcAslButtnOnOffCncl2"
  CcAslButtnOnPress2/1 -> bus_creator/15  "CcAslButtnOnPress2"
  CcAslButtnResDecPress2/1 -> bus_creator/16  "CcAslButtnResDecPress2"
  CcAslButtnResIncPress2/1 -> bus_creator/17  "CcAslButtnResIncPress2"
  CcAslButtnSetDecPress2/1 -> bus_creator/18  "CcAslButtnSetDecPress2"
  CcAslButtnSetIncPress2/1 -> bus_creator/19  "CcAslButtnSetIncPress2"
  CcAslButtnSetPress2/1 -> bus_creator/20  "CcAslButtnSetPress2"
  CcAsllButtnResPress2/1 -> bus_creator/21  "CcAsllButtnResPress2"
  CcButtnOffPress2/1 -> bus_creator/22  "CcButtnOffPress2"
  CcButtnOnOffCnclPress2/1 -> bus_creator/23  "CcButtnOnOffCnclPress2"
  CcButtnOnOffPress2/1 -> bus_creator/24  "CcButtnOnOffPress2"
  CcButtnOnPress2/1 -> bus_creator/25  "CcButtnOnPress2"
  SelDrvMdeAdptSte_D_Stat/1 -> bus_creator/26  "SelDrvMdeAdptSte_D_Stat"
  TjaButtnOnOffPress2/1 -> bus_creator/27  "TjaButtnOnOffPress2"

== system P702_NI_SoftECU/Output/Subsystem2/CAN_Signal/GWM/Other_GWMTx/DCACA_Data1_FD1 ==
  CoolFanDcac_D_Rq : Constant  Value=0
  DcacClntFlw_D_Rq : Constant  Value=0
  DcacPlugPrsnt_B_Stat : Constant  Value=0
  DcacRdy_D_Stat : Constant  Value=0
  bus_creator : BusCreator  Inputs=4
  out_port : Outport
  wires:
  bus_creator/1 -> out_port/1  "Subsystem2"
  CoolFanDcac_D_Rq/1 -> bus_creator/1  "CoolFanDcac_D_Rq"
  DcacClntFlw_D_Rq/1 -> bus_creator/2  "DcacClntFlw_D_Rq"
  DcacPlugPrsnt_B_Stat/1 -> bus_creator/3  "DcacPlugPrsnt_B_Stat"
  DcacRdy_D_Stat/1 -> bus_creator/4  "DcacRdy_D_Stat"

== system P702_NI_SoftECU/Output/Subsystem2/CAN_Signal/GWM/Other_GWMTx/DCACA_Data2_FD1 ==
  DcacIn_I_Actl : Constant  Value=0
  DcacIn_U_Actl : Constant  Value=0
  Dcac_Te_Actl : Constant  Value=0
  bus_creator : BusCreator  Inputs=3
  out_port : Outport
  wires:
  bus_creator/1 -> out_port/1  "Subsystem2"
  DcacIn_I_Actl/1 -> bus_creator/1  "DcacIn_I_Actl"
  DcacIn_U_Actl/1 -> bus_creator/2  "DcacIn_U_Actl"
  Dcac_Te_Actl/1 -> bus_creator/3  "Dcac_Te_Actl"

== system P702_NI_SoftECU/Output/Subsystem2/CAN_Signal/GWM/Other_GWMTx/DCACA_Data3_FD1 ==
  DcacIn_Pw_Mx : Constant  Value=0
  DcacOut1_Pw_Actl : Constant  Value=0
  DcacOut2_Pw_Actl : Constant  Value=0
  DcacOut_Pw_Mx : Constant  Value=0
  bus_creator : BusCreator  Inputs=4
  out_port : Outport
  wires:
  bus_creator/1 -> out_port/1  "Subsystem2"
  DcacIn_Pw_Mx/1 -> bus_creator/1  "DcacIn_Pw_Mx"
  DcacOut1_Pw_Actl/1 -> bus_creator/2  "DcacOut1_Pw_Actl"
  DcacOut2_Pw_Actl/1 -> bus_creator/3  "DcacOut2_Pw_Actl"
  DcacOut_Pw_Mx/1 -> bus_creator/4  "DcacOut_Pw_Mx"

== system P702_NI_SoftECU/Output/Subsystem2/CAN_Signal/GWM/Other_GWMTx/DifferentialCtrlData_1_FD1 ==
  RearDiffLck_Tq_Actl2 : Constant  Value=0
  bus_creator : BusCreator  Inputs=1
  out_port : Outport
  wires:
  bus_creator/1 -> out_port/1  "Subsystem2"
  RearDiffLck_Tq_Actl2/1 -> bus_creator/1  "RearDiffLck_Tq_Actl2"

== system P702_NI_SoftECU/Output/Subsystem2/CAN_Signal/GWM/Other_GWMTx/Driver_Dr_Stat_FD1 ==
  BLISLEDStatDriverSide : Constant  Value=0
  ChildLckFdbckRd_B_Stat : Constant  Value=0
  ChildLckPw_D_Rq : Constant  Value=0
  ChildLckPw_N_Cnt : Constant  Value=0
  Driver_Lock_Sw_Cnt : Constant  Value=0
  Driver_Lock_Sw_Stat : Constant  Value=0
  KeyCylSwDrvDr_D_Stat : Constant  Value=0
  RollCodeDrvDrKeyCyl : Constant  Value=0
  RvrseMirrorChime_B_Rq : Constant  Value=0
  WndwDrvSide_D_Stat : Constant  Value=0
  bus_creator : BusCreator  Inputs=10
  out_port : Outport
  wires:
  bus_creator/1 -> out_port/1  "Subsystem2"
  BLISLEDStatDriverSide/1 -> bus_creator/1  "BLISLEDStatDriverSide"
  ChildLckFdbckRd_B_Stat/1 -> bus_creator/2  "ChildLckFdbckRd_B_Stat"
  ChildLckPw_D_Rq/1 -> bus_creator/3  "ChildLckPw_D_Rq"
  ChildLckPw_N_Cnt/1 -> bus_creator/4  "ChildLckPw_N_Cnt"
  Driver_Lock_Sw_Cnt/1 -> bus_creator/5  "Driver_Lock_Sw_Cnt"
  Driver_Lock_Sw_Stat/1 -> bus_creator/6  "Driver_Lock_Sw_Stat"
  KeyCylSwDrvDr_D_Stat/1 -> bus_creator/7  "KeyCylSwDrvDr_D_Stat"
  RollCodeDrvDrKeyCyl/1 -> bus_creator/8  "RollCodeDrvDrKeyCyl"
  RvrseMirrorChime_B_Rq/1 -> bus_creator/9  "RvrseMirrorChime_B_Rq"
  WndwDrvSide_D_Stat/1 -> bus_creator/10  "WndwDrvSide_D_Stat"

== system P702_NI_SoftECU/Output/Subsystem2/CAN_Signal/GWM/Other_GWMTx/Dsp_Request_Signals11_FD1 ==
  ApaMdeStat_D_RqDrv : Constant  Value=0
  ApaSwtch_D_RqMnu : Constant  Value=0
  CamAutoTowbarZoom : Constant  Value=0
  CamraOvrlDyn_D_Rq : Constant  Value=0
  CamraOvrlStat_D_Rq : Constant  Value=0
  CamraViewSplit_B_Rq : Constant  Value=0
  CamraZoomMan_D_Rq : Constant  Value=0
  DistanceBarSetting : Constant  Value=0
  PrkAidSwtch_D_RqMnu : Constant  Value=0
  bus_creator : BusCreator  Inputs=9
  out_port : Outport
  wires:
  bus_creator/1 -> out_port/1  "Subsystem2"
  ApaMdeStat_D_RqDrv/1 -> bus_creator/1  "ApaMdeStat_D_RqDrv"
  ApaSwtch_D_RqMnu/1 -> bus_creator/2  "ApaSwtch_D_RqMnu"
  CamAutoTowbarZoom/1 -> bus_creator/3  "CamAutoTowbarZoom"
  CamraOvrlDyn_D_Rq/1 -> bus_creator/4  "CamraOvrlDyn_D_Rq"
  CamraOvrlStat_D_Rq/1 -> bus_creator/5  "CamraOvrlStat_D_Rq"
  CamraViewSplit_B_Rq/1 -> bus_creator/6  "CamraViewSplit_B_Rq"
  CamraZoomMan_D_Rq/1 -> bus_creator/7  "CamraZoomMan_D_Rq"
  DistanceBarSetting/1 -> bus_creator/8  "DistanceBarSetting"
  PrkAidSwtch_D_RqMnu/1 -> bus_creator/9  "PrkAidSwtch_D_RqMnu"

== system P702_NI_SoftECU/Output/Subsystem2/CAN_Signal/GWM/Other_GWMTx/ElecHorizon_Data1_FD1 ==
  EhData1_No_Actl : Constant  Value=0
  bus_creator : BusCreator  Inputs=1
  out_port : Outport
  wires:
  bus_creator/1 -> out_port/1  "Subsystem2"
  EhData1_No_Actl/1 -> bus_creator/1  "EhData1_No_Actl"

== system P702_NI_SoftECU/Output/Subsystem2/CAN_Signal/GWM/Other_GWMTx/ElecHorizon_Data2_FD1 ==
  EhData2_No_Actl : Constant  Value=0
  bus_creator : BusCreator  Inputs=1
  out_port : Outport
  wires:
  bus_creator/1 -> out_port/1  "Subsystem2"
  EhData2_No_Actl/1 -> bus_creator/1  "EhData2_No_Actl"

== system P702_NI_SoftECU/Output/Subsystem2/CAN_Signal/GWM/Other_GWMTx/FourByFourSwitchData_FD1 ==
  AwdLck_D_RqDrv : Constant  Value=0
  AwdMde_D_RqDrv : Constant  Value=0
  DrvSlipCtlMde_B_Rq3 : Constant  Value=0
  HdcSwtchPos_B_Actl : Constant  Value=0
  HybMdeSwtch_B_Rq : Constant  Value=0
  RearDiffLck_D_RqDrv : Constant  Value=0
  TrailCtlSwtch_B_Stat3 : Constant  Value=0
  bus_creator : BusCreator  Inputs=7
  out_port : Outport
  wires:
  bus_creator/1 -> out_port/1  "Subsystem2"
  AwdLck_D_RqDrv/1 -> bus_creator/1  "AwdLck_D_RqDrv"
  AwdMde_D_RqDrv/1 -> bus_creator/2  "AwdMde_D_RqDrv"
  DrvSlipCtlMde_B_Rq3/1 -> bus_creator/3  "DrvSlipCtlMde_B_Rq3"
  HdcSwtchPos_B_Actl/1 -> bus_creator/4  "HdcSwtchPos_B_Actl"
  HybMdeSwtch_B_Rq/1 -> bus_creator/5  "HybMdeSwtch_B_Rq"
  RearDiffLck_D_RqDrv/1 -> bus_creator/6  "RearDiffLck_D_RqDrv"
  TrailCtlSwtch_B_Stat3/1 -> bus_creator/7  "TrailCtlSwtch_B_Stat3"

== system P702_NI_SoftECU/Output/Subsystem2/CAN_Signal/GWM/Other_GWMTx/Front_Distance_Req_FD1 ==
  FdsmTrgCntr_B_Actl : Constant  Value=0
  FdsmTrgDist_L_Actl : Constant  Value=0
  FdsmTrgLeft_B_Actl : Constant  Value=0
  FdsmTrgRight_B_Actl : Constant  Value=0
  LscmbbBaSens_D_Rq : Constant  Value=0
  LscmbbBlck_B_Actl : Constant  Value=0
  LscmbbBrkDecel_A_Rq : Constant  Value=0
  LscmbbBrkDecel_B_Enbl : Constant  Value=0
  LscmbbBrkDecel_No_Cnt : Constant  Value=0
  LscmbbBrkDecel_No_Cs : Constant  Value=0
  LscmbbBrkPrchg_D_Rq : Constant  Value=0
  LscmbbDeny_B_Actl : Constant  Value=0
  LscmbbEngTqMn_B_Rq : Constant  Value=0
  LscmbbMsgTxt_D_Rq : Constant  Value=0
  LscmbbPostEvnt_B_Dsply : Constant  Value=0
  LscmbbSrvcRqd_B_Rq : Constant  Value=0
  WndwFrontHeat_B_Rq : Constant  Value=0
  bus_creator : BusCreator  Inputs=17
  out_port : Outport
  wires:
  bus_creator/1 -> out_port/1  "Subsystem2"
  FdsmTrgCntr_B_Actl/1 -> bus_creator/1  "FdsmTrgCntr_B_Actl"
  FdsmTrgDist_L_Actl/1 -> bus_creator/2  "FdsmTrgDist_L_Actl"
  FdsmTrgLeft_B_Actl/1 -> bus_creator/3  "FdsmTrgLeft_B_Actl"
  FdsmTrgRight_B_Actl/1 -> bus_creator/4  "FdsmTrgRight_B_Actl"
  LscmbbBaSens_D_Rq/1 -> bus_creator/5  "LscmbbBaSens_D_Rq"
  LscmbbBlck_B_Actl/1 -> bus_creator/6  "LscmbbBlck_B_Actl"
  LscmbbBrkDecel_A_Rq/1 -> bus_creator/7  "LscmbbBrkDecel_A_Rq"
  LscmbbBrkDecel_B_Enbl/1 -> bus_creator/8  "LscmbbBrkDecel_B_Enbl"
  LscmbbBrkDecel_No_Cnt/1 -> bus_creator/9  "LscmbbBrkDecel_No_Cnt"
  LscmbbBrkDecel_No_Cs/1 -> bus_creator/10  "LscmbbBrkDecel_No_Cs"
  LscmbbBrkPrchg_D_Rq/1 -> bus_creator/11  "LscmbbBrkPrchg_D_Rq"
  LscmbbDeny_B_Actl/1 -> bus_creator/12  "LscmbbDeny_B_Actl"
  LscmbbEngTqMn_B_Rq/1 -> bus_creator/13  "LscmbbEngTqMn_B_Rq"
  LscmbbMsgTxt_D_Rq/1 -> bus_creator/14  "LscmbbMsgTxt_D_Rq"
  LscmbbPostEvnt_B_Dsply/1 -> bus_creator/15  "LscmbbPostEvnt_B_Dsply"
  LscmbbSrvcRqd_B_Rq/1 -> bus_creator/16  "LscmbbSrvcRqd_B_Rq"
  WndwFrontHeat_B_Rq/1 -> bus_creator/17  "WndwFrontHeat_B_Rq"

== system P702_NI_SoftECU/Output/Subsystem2/CAN_Signal/GWM/Other_GWMTx/GGCC_Config_Mgmt_ID_1_FD1 ==
  VehicleGGCCData : Constant  Value=0
  bus_creator : BusCreator  Inputs=1
  out_port : Outport
  wires:
  bus_creator/1 -> out_port/1  "Subsystem2"
  VehicleGGCCData/1 -> bus_creator/1  "VehicleGGCCData"

== system P702_NI_SoftECU/Output/Subsystem2/CAN_Signal/GWM/Other_GWMTx/GWM_AutoSar_NetMgmt_FD1 ==
  GWM_AutoSarNMControl : Constant  Value=0
  GWM_AutoSarNMNodeId : Constant  Value=0
  GWM_AutoSarNMReserved{1..4} (4 alike) : Constant  Value=0
  GWM_GWNMProxy : Constant  Value=0
  GWM_GWOnBoardTester : Constant  Value=0
  bus_creator : BusCreator  Inputs=8
  out_port : Outport
  wires:
  bus_creator/1 -> out_port/1  "Subsystem2"
  GWM_AutoSarNMControl/1 -> bus_creator/1  "GWM_AutoSarNMControl"
  GWM_AutoSarNMNodeId/1 -> bus_creator/2  "GWM_AutoSarNMNodeId"
  GWM_AutoSarNMReserved1/1 -> bus_creator/3  "GWM_AutoSarNMReserved1"
  GWM_AutoSarNMReserved2/1 -> bus_creator/4  "GWM_AutoSarNMReserved2"
  GWM_AutoSarNMReserved3/1 -> bus_creator/5  "GWM_AutoSarNMReserved3"
  GWM_AutoSarNMReserved4/1 -> bus_creator/6  "GWM_AutoSarNMReserved4"
  GWM_GWNMProxy/1 -> bus_creator/7  "GWM_GWNMProxy"
  GWM_GWOnBoardTester/1 -> bus_creator/8  "GWM_GWOnBoardTester"

== system P702_NI_SoftECU/Output/Subsystem2/CAN_Signal/GWM/Other_GWMTx/GlobalClock_Data_FD1 ==
  GlblClkDay_No_Actl : Constant  Value=0
  GlblClkHr_No_Actl : Constant  Value=0
  GlblClkMnte_No_Actl : Constant  Value=0
  GlblClkScnd_No_Actl : Constant  Value=0
  GlblClkYr_No_Actl : Constant  Value=0
  bus_creator : BusCreator  Inputs=5
  out_port : Outport
  wires:
  bus_creator/1 -> out_port/1  "Subsystem2"
  GlblClkDay_No_Actl/1 -> bus_creator/1  "GlblClkDay_No_Actl"
  GlblClkHr_No_Actl/1 -> bus_creator/2  "GlblClkHr_No_Actl"
  GlblClkMnte_No_Actl/1 -> bus_creator/3  "GlblClkMnte_No_Actl"
  GlblClkScnd_No_Actl/1 -> bus_creator/4  "GlblClkScnd_No_Actl"
  GlblClkYr_No_Actl/1 -> bus_creator/5  "GlblClkYr_No_Actl"

== system P702_NI_SoftECU/Output/Subsystem2/CAN_Signal/GWM/Other_GWMTx/Global_PATS_Cntrl_Info_FD1 ==
  bus_creator : BusCreator  Inputs=2
  immoControlCmd_T1 : Constant  Value=0
  immoControlData_T1 : Constant  Value=0
  out_port : Outport
  wires:
  bus_creator/1 -> out_port/1  "Subsystem2"
  immoControlCmd_T1/1 -> bus_creator/1  "immoControlCmd_T1"
  immoControlData_T1/1 -> bus_creator/2  "immoControlData_T1"

== system P702_NI_SoftECU/Output/Subsystem2/CAN_Signal/GWM/Other_GWMTx/IPC_Infotainment_FD1 ==
  BeltminderAudioMute : Constant  Value=0
  Chime_Source : Constant  Value=0
  HdcOn_B_Rq : Constant  Value=0
  IPC_Attn_Info_Audio : Constant  Value=0
  IPC_MyKeyVolLimit_St : Constant  Value=0
  IPC_New_Attn_Event : Constant  Value=0
  Power_Up_Chime_Modules : Constant  Value=0
  Veh_V2_Dsply : Constant  Value=0
  bus_creator : BusCreator  Inputs=8
  out_port : Outport
  wires:
  bus_creator/1 -> out_port/1  "Subsystem2"
  BeltminderAudioMute/1 -> bus_creator/1  "BeltminderAudioMute"
  Chime_Source/1 -> bus_creator/2  "Chime_Source"
  HdcOn_B_Rq/1 -> bus_creator/3  "HdcOn_B_Rq"
  IPC_Attn_Info_Audio/1 -> bus_creator/4  "IPC_Attn_Info_Audio"
  IPC_MyKeyVolLimit_St/1 -> bus_creator/5  "IPC_MyKeyVolLimit_St"
  IPC_New_Attn_Event/1 -> bus_creator/6  "IPC_New_Attn_Event"
  Power_Up_Chime_Modules/1 -> bus_creator/7  "Power_Up_Chime_Modules"
  Veh_V2_Dsply/1 -> bus_creator/8  "Veh_V2_Dsply"

== system P702_NI_SoftECU/Output/Subsystem2/CAN_Signal/GWM/Other_GWMTx/IPC_Send_Signals_2_FD1 ==
  ElLongTerm_L_Dsply : Constant  Value=0
  ElTrip_L_Dsply : Constant  Value=0
  FuelRange_L_Dsply : Constant  Value=0
  bus_creator : BusCreator  Inputs=3
  out_port : Outport
  wires:
  bus_creator/1 -> out_port/1  "Subsystem2"
  ElLongTerm_L_Dsply/1 -> bus_creator/1  "ElLongTerm_L_Dsply"
  ElTrip_L_Dsply/1 -> bus_creator/2  "ElTrip_L_Dsply"
  FuelRange_L_Dsply/1 -> bus_creator/3  "FuelRange_L_Dsply"

== system P702_NI_SoftECU/Output/Subsystem2/CAN_Signal/GWM/Other_GWMTx/MHT_EV_Wakeup_FD1 ==
  BattChlrSov_B_Rq : Constant  Value=0
  BattChrgTrgtSoC_D_Rq : Constant  Value=0
  BattTracDrvSustn_B_Rq : Constant  Value=0
  BrkAppl_D_RqPt : Constant  Value=0
  CabnEvapSovFront_B_Rq : Constant  Value=0
  CabnEvapSovRear_B_Rq : Constant  Value=0
  HeatCoreSovRear_B_Rq : Constant  Value=0
  HtrnClntFlw_D_Rq : Constant  Value=0
  HtrnCnnctPwr_B_Stat : Constant  Value=0
  HtrnDcdcDis_B_Rq : Constant  Value=0
  PtcHtr_D_Stat : Constant  Value=0
  bus_creator : BusCreator  Inputs=11
  out_port : Outport
  wires:
  bus_creator/1 -> out_port/1  "Subsystem2"
  BattChlrSov_B_Rq/1 -> bus_creator/1  "BattChlrSov_B_Rq"
  BattChrgTrgtSoC_D_Rq/1 -> bus_creator/2  "BattChrgTrgtSoC_D_Rq"
  BattTracDrvSustn_B_Rq/1 -> bus_creator/3  "BattTracDrvSustn_B_Rq"
  BrkAppl_D_RqPt/1 -> bus_creator/4  "BrkAppl_D_RqPt"
  CabnEvapSovFront_B_Rq/1 -> bus_creator/5  "CabnEvapSovFront_B_Rq"
  CabnEvapSovRear_B_Rq/1 -> bus_creator/6  "CabnEvapSovRear_B_Rq"
  HeatCoreSovRear_B_Rq/1 -> bus_creator/7  "HeatCoreSovRear_B_Rq"
  HtrnClntFlw_D_Rq/1 -> bus_creator/8  "HtrnClntFlw_D_Rq"
  HtrnCnnctPwr_B_Stat/1 -> bus_creator/9  "HtrnCnnctPwr_B_Stat"
  HtrnDcdcDis_B_Rq/1 -> bus_creator/10  "HtrnDcdcDis_B_Rq"
  PtcHtr_D_Stat/1 -> bus_creator/11  "PtcHtr_D_Stat"

== system P702_NI_SoftECU/Output/Subsystem2/CAN_Signal/GWM/Other_GWMTx/Mc_Send_Signals_2_FD1 ==
  BttOn_B_Rq : Constant  Value=0
  Btt_L_Actl : Constant  Value=0
  EngExhMdeQuiet_D_Rq : Constant  Value=0
  EsaOn_B_Rq : Constant  Value=0
  Mc_VehLangUsrSel_St : Constant  Value=0
  Mc_VehUnitTempUsrSel_St : Constant  Value=0
  Mc_VehUntTrpCoUsrSel_St : Constant  Value=0
  SelDrvMdeDsply_B_Avail : Constant  Value=0
  SelDrvMdeTxtReset_B_Rq : Constant  Value=0
  WaitToStartLamp_D_Falt : Constant  Value=0
  bus_creator : BusCreator  Inputs=10
  out_port : Outport
  wires:
  bus_creator/1 -> out_port/1  "Subsystem2"
  BttOn_B_Rq/1 -> bus_creator/1  "BttOn_B_Rq"
  Btt_L_Actl/1 -> bus_creator/2  "Btt_L_Actl"
  EngExhMdeQuiet_D_Rq/1 -> bus_creator/3  "EngExhMdeQuiet_D_Rq"
  EsaOn_B_Rq/1 -> bus_creator/4  "EsaOn_B_Rq"
  Mc_VehLangUsrSel_St/1 -> bus_creator/5  "Mc_VehLangUsrSel_St"
  Mc_VehUnitTempUsrSel_St/1 -> bus_creator/6  "Mc_VehUnitTempUsrSel_St"
  Mc_VehUntTrpCoUsrSel_St/1 -> bus_creator/7  "Mc_VehUntTrpCoUsrSel_St"
  SelDrvMdeDsply_B_Avail/1 -> bus_creator/8  "SelDrvMdeDsply_B_Avail"
  SelDrvMdeTxtReset_B_Rq/1 -> bus_creator/9  "SelDrvMdeTxtReset_B_Rq"
  WaitToStartLamp_D_Falt/1 -> bus_creator/10  "WaitToStartLamp_D_Falt"

== system P702_NI_SoftECU/Output/Subsystem2/CAN_Signal/GWM/Other_GWMTx/ParkAid_Aud_Warn_CmdM_FD1 ==
  Cta_D_Rq : Constant  Value=0
  PrkAidRear_D_RqDrv : Constant  Value=0
  Sod_D_Rq : Constant  Value=0
  SteEffort_D_Rq : Constant  Value=0
  bus_creator : BusCreator  Inputs=4
  out_port : Outport
  wires:
  bus_creator/1 -> out_port/1  "Subsystem2"
  Cta_D_Rq/1 -> bus_creator/1  "Cta_D_Rq"
  PrkAidRear_D_RqDrv/1 -> bus_creator/2  "PrkAidRear_D_RqDrv"
  Sod_D_Rq/1 -> bus_creator/3  "Sod_D_Rq"
  SteEffort_D_Rq/1 -> bus_creator/4  "SteEffort_D_Rq"

== system P702_NI_SoftECU/Output/Subsystem2/CAN_Signal/GWM/Other_GWMTx/Pass_Dr_Stat_FD1 ==
  BLISLEDStatPassSide : Constant  Value=0
  ChildLckFdbckRp_B_Stat : Constant  Value=0
  Memory_1_SwPsngr_Stat : Constant  Value=0
  Memory_2_SwPsngr_Stat : Constant  Value=0
  Memory_3_SwPsngr_Stat : Constant  Value=0
  Pasngr_Lock_Sw_Cnt : Constant  Value=0
  Pasngr_Lock_Sw_Stat : Constant  Value=0
  RollCode_No_ActlPdm : Constant  Value=0
  WndwPsngrSide_D_Stat : Constant  Value=0
  bus_creator : BusCreator  Inputs=9
  out_port : Outport
  wires:
  bus_creator/1 -> out_port/1  "Subsystem2"
  BLISLEDStatPassSide/1 -> bus_creator/1  "BLISLEDStatPassSide"
  ChildLckFdbckRp_B_Stat/1 -> bus_creator/2  "ChildLckFdbckRp_B_Stat"
  Memory_1_SwPsngr_Stat/1 -> bus_creator/3  "Memory_1_SwPsngr_Stat"
  Memory_2_SwPsngr_Stat/1 -> bus_creator/4  "Memory_2_SwPsngr_Stat"
  Memory_3_SwPsngr_Stat/1 -> bus_creator/5  "Memory_3_SwPsngr_Stat"
  Pasngr_Lock_Sw_Cnt/1 -> bus_creator/6  "Pasngr_Lock_Sw_Cnt"
  Pasngr_Lock_Sw_Stat/1 -> bus_creator/7  "Pasngr_Lock_Sw_Stat"
  RollCode_No_ActlPdm/1 -> bus_creator/8  "RollCode_No_ActlPdm"
  WndwPsngrSide_D_Stat/1 -> bus_creator/9  "WndwPsngrSide_D_Stat"

== system P702_NI_SoftECU/Output/Subsystem2/CAN_Signal/GWM/Other_GWMTx/Personality_APIM_Data_FD1 ==
  CtrStkDsplyOp_D_Rq : Constant  Value=0
  CtrStkFeatConfigActl : Constant  Value=0
  CtrStkFeatNoActl : Constant  Value=0
  CtrStkPersIndex_D_Actl : Constant  Value=0
  Pers1OptIn_B_Stats : Constant  Value=0
  Pers2OptIn_B_Stats : Constant  Value=0
  Pers3OptIn_B_Stats : Constant  Value=0
  Pers4OptIn_B_Stats : Constant  Value=0
  PersStore_D_Rq : Constant  Value=0
  bus_creator : BusCreator  Inputs=9
  out_port : Outport
  wires:
  bus_creator/1 -> out_port/1  "Subsystem2"
  CtrStkDsplyOp_D_Rq/1 -> bus_creator/1  "CtrStkDsplyOp_D_Rq"
  CtrStkFeatConfigActl/1 -> bus_creator/2  "CtrStkFeatConfigActl"
  CtrStkFeatNoActl/1 -> bus_creator/3  "CtrStkFeatNoActl"
  CtrStkPersIndex_D_Actl/1 -> bus_creator/4  "CtrStkPersIndex_D_Actl"
  Pers1OptIn_B_Stats/1 -> bus_creator/5  "Pers1OptIn_B_Stats"
  Pers2OptIn_B_Stats/1 -> bus_creator/6  "Pers2OptIn_B_Stats"
  Pers3OptIn_B_Stats/1 -> bus_creator/7  "Pers3OptIn_B_Stats"
  Pers4OptIn_B_Stats/1 -> bus_creator/8  "Pers4OptIn_B_Stats"
  PersStore_D_Rq/1 -> bus_creator/9  "PersStore_D_Rq"

== system P702_NI_SoftECU/Output/Subsystem2/CAN_Signal/GWM/Other_GWMTx/Personality_Data_FD1 ==
  MsgCntrDsplyOp_D_Rq : Constant  Value=0
  MsgCntrFeatConfigRq : Constant  Value=0
  MsgCntrFeatNoRq : Constant  Value=0
  MsgCntrPersIndex_D_Rq : Constant  Value=0
  bus_creator : BusCreator  Inputs=4
  out_port : Outport
  wires:
  bus_creator/1 -> out_port/1  "Subsystem2"
  MsgCntrDsplyOp_D_Rq/1 -> bus_creator/1  "MsgCntrDsplyOp_D_Rq"
  MsgCntrFeatConfigRq/1 -> bus_creator/2  "MsgCntrFeatConfigRq"
  MsgCntrFeatNoRq/1 -> bus_creator/3  "MsgCntrFeatNoRq"
  MsgCntrPersIndex_D_Rq/1 -> bus_creator/4  "MsgCntrPersIndex_D_Rq"
